simulink model "modelWithSimscapeRobotAndEnvironmentDynamics"  (R2020b)
settings: Solver=daessc  StartTime=0.0  StopTime=16  MaxStep=0.1  RelTol=1e-2  AbsTol=1e-2
values from neighbouring files (symbols this model uses):
  dq0 = zeros(size(q0))    [RobotTest.m]
  N = size(jointLim, 1)    [robotIK.m]
  q0 = homeConfiguration(lbr)    [MKC.m]    (also in RobotTest.m = configSequence(:,1))
  widgetDimensions = [0.02 0.02 0.07]    [RobotTest.m]
undefined symbols (not defined in the file or in its folder): CenterTable, configSequence, Floor, LeftShelf, X, Y, Z
libraries: sm_lib x273, nesl_utility x75, robotmaniplib x3, robotcorelib x1
(part 2 of 7)

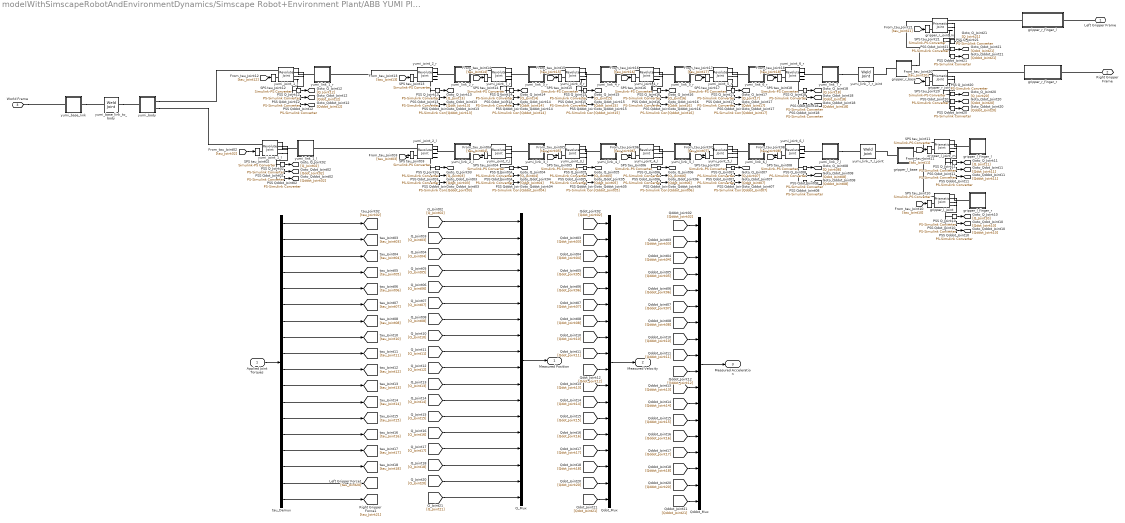
== system modelWithSimscapeRobotAndEnvironmentDynamics/Simscape Robot+Environment Plant/ABB YUMI Plant Model ==
  Applied Joint Torques : Inport
  PSS Q_Joint02 : nesl_utility/PS-Simulink Converter  PhysicalDomain=network_engine_domain  SubClassName=ps_output  LeftPortType=input  RightPortType=output  PseudoPeriodic=off  Frequencies=[]  Unit=inherit  AffineConversion=off
      settings: SourceProductName=Utilities
  PSS Q_Joint03 : nesl_utility/PS-Simulink Converter  PhysicalDomain=network_engine_domain  SubClassName=ps_output  LeftPortType=input  RightPortType=output  PseudoPeriodic=off  Frequencies=[]  Unit=inherit  AffineConversion=off
      settings: SourceProductName=Utilities
  PSS Q_Joint04 : nesl_utility/PS-Simulink Converter  PhysicalDomain=network_engine_domain  SubClassName=ps_output  LeftPortType=input  RightPortType=output  PseudoPeriodic=off  Frequencies=[]  Unit=inherit  AffineConversion=off
      settings: SourceProductName=Utilities
  PSS Q_Joint05 : nesl_utility/PS-Simulink Converter  PhysicalDomain=network_engine_domain  SubClassName=ps_output  LeftPortType=input  RightPortType=output  PseudoPeriodic=off  Frequencies=[]  Unit=inherit  AffineConversion=off
      settings: SourceProductName=Utilities
  PSS Q_Joint06 : nesl_utility/PS-Simulink Converter  PhysicalDomain=network_engine_domain  SubClassName=ps_output  LeftPortType=input  RightPortType=output  PseudoPeriodic=off  Frequencies=[]  Unit=inherit  AffineConversion=off
      settings: SourceProductName=Utilities
  PSS Q_Joint07 : nesl_utility/PS-Simulink Converter  PhysicalDomain=network_engine_domain  SubClassName=ps_output  LeftPortType=input  RightPortType=output  PseudoPeriodic=off  Frequencies=[]  Unit=inherit  AffineConversion=off
      settings: SourceProductName=Utilities
  PSS Q_Joint08 : nesl_utility/PS-Simulink Converter  PhysicalDomain=network_engine_domain  SubClassName=ps_output  LeftPortType=input  RightPortType=output  PseudoPeriodic=off  Frequencies=[]  Unit=inherit  AffineConversion=off
      settings: SourceProductName=Utilities
  PSS Q_Joint{10..18,20..21} (11 alike) : nesl_utility/PS-Simulink Converter  PhysicalDomain=network_engine_domain  SubClassName=ps_output  LeftPortType=input  RightPortType=output  PseudoPeriodic=off  Frequencies=[]  Unit=inherit  AffineConversion=off
      settings: SourceProductName=Utilities
  PSS Qddot_Joint02 : nesl_utility/PS-Simulink Converter  PhysicalDomain=network_engine_domain  SubClassName=ps_output  LeftPortType=input  RightPortType=output  PseudoPeriodic=off  Frequencies=[]  Unit=inherit  AffineConversion=off
      settings: SourceProductName=Utilities
  PSS Qddot_Joint03 : nesl_utility/PS-Simulink Converter  PhysicalDomain=network_engine_domain  SubClassName=ps_output  LeftPortType=input  RightPortType=output  PseudoPeriodic=off  Frequencies=[]  Unit=inherit  AffineConversion=off
      settings: SourceProductName=Utilities
  PSS Qddot_Joint04 : nesl_utility/PS-Simulink Converter  PhysicalDomain=network_engine_domain  SubClassName=ps_output  LeftPortType=input  RightPortType=output  PseudoPeriodic=off  Frequencies=[]  Unit=inherit  AffineConversion=off
      settings: SourceProductName=Utilities
  PSS Qddot_Joint05 : nesl_utility/PS-Simulink Converter  PhysicalDomain=network_engine_domain  SubClassName=ps_output  LeftPortType=input  RightPortType=output  PseudoPeriodic=off  Frequencies=[]  Unit=inherit  AffineConversion=off
      settings: SourceProductName=Utilities
  PSS Qddot_Joint06 : nesl_utility/PS-Simulink Converter  PhysicalDomain=network_engine_domain  SubClassName=ps_output  LeftPortType=input  RightPortType=output  PseudoPeriodic=off  Frequencies=[]  Unit=inherit  AffineConversion=off
      settings: SourceProductName=Utilities
  PSS Qddot_Joint07 : nesl_utility/PS-Simulink Converter  PhysicalDomain=network_engine_domain  SubClassName=ps_output  LeftPortType=input  RightPortType=output  PseudoPeriodic=off  Frequencies=[]  Unit=inherit  AffineConversion=off
      settings: SourceProductName=Utilities
  PSS Qddot_Joint08 : nesl_utility/PS-Simulink Converter  PhysicalDomain=network_engine_domain  SubClassName=ps_output  LeftPortType=input  RightPortType=output  PseudoPeriodic=off  Frequencies=[]  Unit=inherit  AffineConversion=off
      settings: SourceProductName=Utilities
  PSS Qddot_Joint{10..18,20..21} (11 alike) : nesl_utility/PS-Simulink Converter  PhysicalDomain=network_engine_domain  SubClassName=ps_output  LeftPortType=input  RightPortType=output  PseudoPeriodic=off  Frequencies=[]  Unit=inherit  AffineConversion=off
      settings: SourceProductName=Utilities
  PSS Qdot_Joint02 : nesl_utility/PS-Simulink Converter  PhysicalDomain=network_engine_domain  SubClassName=ps_output  LeftPortType=input  RightPortType=output  PseudoPeriodic=off  Frequencies=[]  Unit=inherit  AffineConversion=off
      settings: SourceProductName=Utilities
  PSS Qdot_Joint03 : nesl_utility/PS-Simulink Converter  PhysicalDomain=network_engine_domain  SubClassName=ps_output  LeftPortType=input  RightPortType=output  PseudoPeriodic=off  Frequencies=[]  Unit=inherit  AffineConversion=off
      settings: SourceProductName=Utilities
  PSS Qdot_Joint04 : nesl_utility/PS-Simulink Converter  PhysicalDomain=network_engine_domain  SubClassName=ps_output  LeftPortType=input  RightPortType=output  PseudoPeriodic=off  Frequencies=[]  Unit=inherit  AffineConversion=off
      settings: SourceProductName=Utilities
  PSS Qdot_Joint05 : nesl_utility/PS-Simulink Converter  PhysicalDomain=network_engine_domain  SubClassName=ps_output  LeftPortType=input  RightPortType=output  PseudoPeriodic=off  Frequencies=[]  Unit=inherit  AffineConversion=off
      settings: SourceProductName=Utilities
  PSS Qdot_Joint06 : nesl_utility/PS-Simulink Converter  PhysicalDomain=network_engine_domain  SubClassName=ps_output  LeftPortType=input  RightPortType=output  PseudoPeriodic=off  Frequencies=[]  Unit=inherit  AffineConversion=off
      settings: SourceProductName=Utilities
  PSS Qdot_Joint07 : nesl_utility/PS-Simulink Converter  PhysicalDomain=network_engine_domain  SubClassName=ps_output  LeftPortType=input  RightPortType=output  PseudoPeriodic=off  Frequencies=[]  Unit=inherit  AffineConversion=off
      settings: SourceProductName=Utilities
  PSS Qdot_Joint08 : nesl_utility/PS-Simulink Converter  PhysicalDomain=network_engine_domain  SubClassName=ps_output  LeftPortType=input  RightPortType=output  PseudoPeriodic=off  Frequencies=[]  Unit=inherit  AffineConversion=off
      settings: SourceProductName=Utilities
  PSS Qdot_Joint{10..18,20..21} (11 alike) : nesl_utility/PS-Simulink Converter  PhysicalDomain=network_engine_domain  SubClassName=ps_output  LeftPortType=input  RightPortType=output  PseudoPeriodic=off  Frequencies=[]  Unit=inherit  AffineConversion=off
      settings: SourceProductName=Utilities
  Q_Mux : Mux  Inputs=18
  Qddot_Mux : Mux  Inputs=18
  Qdot_Mux : Mux  Inputs=18
  SPS tau_Joint02 : nesl_utility/Simulink-PS Converter  PhysicalDomain=network_engine_domain  SubClassName=ps_input  LeftPortType=input  RightPortType=output  PseudoPeriodic=off  Frequencies=[]  NoiseDistribution=none  NoiseParameters=[]  Unit=1  AffineConversion=off  FilteringAndDerivatives=provide  SimscapeFilterOrder=1  InputFilterTimeConstant=0.001  UdotUserProvided=0
      settings: SourceProductName=Utilities
  SPS tau_Joint03 : nesl_utility/Simulink-PS Converter  PhysicalDomain=network_engine_domain  SubClassName=ps_input  LeftPortType=input  RightPortType=output  PseudoPeriodic=off  Frequencies=[]  NoiseDistribution=none  NoiseParameters=[]  Unit=1  AffineConversion=off  FilteringAndDerivatives=provide  SimscapeFilterOrder=1  InputFilterTimeConstant=0.001  UdotUserProvided=0
      settings: SourceProductName=Utilities
  SPS tau_Joint04 : nesl_utility/Simulink-PS Converter  PhysicalDomain=network_engine_domain  SubClassName=ps_input  LeftPortType=input  RightPortType=output  PseudoPeriodic=off  Frequencies=[]  NoiseDistribution=none  NoiseParameters=[]  Unit=1  AffineConversion=off  FilteringAndDerivatives=provide  SimscapeFilterOrder=1  InputFilterTimeConstant=0.001  UdotUserProvided=0
      settings: SourceProductName=Utilities
  SPS tau_Joint05 : nesl_utility/Simulink-PS Converter  PhysicalDomain=network_engine_domain  SubClassName=ps_input  LeftPortType=input  RightPortType=output  PseudoPeriodic=off  Frequencies=[]  NoiseDistribution=none  NoiseParameters=[]  Unit=1  AffineConversion=off  FilteringAndDerivatives=provide  SimscapeFilterOrder=1  InputFilterTimeConstant=0.001  UdotUserProvided=0
      settings: SourceProductName=Utilities
  SPS tau_Joint06 : nesl_utility/Simulink-PS Converter  PhysicalDomain=network_engine_domain  SubClassName=ps_input  LeftPortType=input  RightPortType=output  PseudoPeriodic=off  Frequencies=[]  NoiseDistribution=none  NoiseParameters=[]  Unit=1  AffineConversion=off  FilteringAndDerivatives=provide  SimscapeFilterOrder=1  InputFilterTimeConstant=0.001  UdotUserProvided=0
      settings: SourceProductName=Utilities
  SPS tau_Joint07 : nesl_utility/Simulink-PS Converter  PhysicalDomain=network_engine_domain  SubClassName=ps_input  LeftPortType=input  RightPortType=output  PseudoPeriodic=off  Frequencies=[]  NoiseDistribution=none  NoiseParameters=[]  Unit=1  AffineConversion=off  FilteringAndDerivatives=provide  SimscapeFilterOrder=1  InputFilterTimeConstant=0.001  UdotUserProvided=0
      settings: SourceProductName=Utilities
  SPS tau_Joint08 : nesl_utility/Simulink-PS Converter  PhysicalDomain=network_engine_domain  SubClassName=ps_input  LeftPortType=input  RightPortType=output  PseudoPeriodic=off  Frequencies=[]  NoiseDistribution=none  NoiseParameters=[]  Unit=1  AffineConversion=off  FilteringAndDerivatives=provide  SimscapeFilterOrder=1  InputFilterTimeConstant=0.001  UdotUserProvided=0
      settings: SourceProductName=Utilities
  SPS tau_Joint{10..18,20..21} (11 alike) : nesl_utility/Simulink-PS Converter  PhysicalDomain=network_engine_domain  SubClassName=ps_input  LeftPortType=input  RightPortType=output  PseudoPeriodic=off  Frequencies=[]  NoiseDistribution=none  NoiseParameters=[]  Unit=1  AffineConversion=off  FilteringAndDerivatives=provide  SimscapeFilterOrder=1  InputFilterTimeConstant=0.001  UdotUserProvided=0
      settings: SourceProductName=Utilities
  gripper_l_base : Subsystem
  gripper_l_finger_l : Subsystem
  gripper_l_finger_r : Subsystem
  gripper_l_joint : sm_lib/Joints/Prismatic Joint  JointMode=Normal  SenseConstraintForce=off  SenseConstraintForceX=off  SenseConstraintForceY=off  SenseConstraintForceZ=off  SenseConstraintTorque=off  SenseConstraintTorqueX=off  SenseConstraintTorqueY=off  SenseConstraintTorqueZ=off  SenseTotalForce=off  SenseTotalForceX=off  SenseTotalForceY=off  SenseTotalForceZ=off  SenseTotalTorque=off  SenseTotalTorqueX=off  SenseTotalTorqueY=off  SenseTotalTorqueZ=off  CompositeWrenchDir=FollowerOnBase  CompositeWrenchFrame=BaseFrame  EquilibriumPosition=0  EquilibriumPositionUnits=m  SpringStiffness=0  SpringStiffnessUnits=N/m  DampingCoefficient=1  DampingCoefficientUnits=kg/s  TorqueActuationMode=InputTorque  MotionActuationMode=ComputedMotion  SensePosition=on  SenseVelocity=on  SenseAcceleration=on  SenseTorqueForce=off  SenseLowerLimitTorqueForce=off  SenseUpperLimitTorqueForce=off  LowerLimitSpecify=on  LowerLimitBound=0  LowerLimitBoundUnits=m  LowerLimitStiffness=1e6  LowerLimitStiffnessUnits=N/m  LowerLimitDamping=1e3  LowerLimitDampingUnits=N/(m/s)  LowerLimitTransitionRegionWidth=1e-4  LowerLimitTransitionRegionWidthUnits=m  UpperLimitSpecify=on  UpperLimitBound=0.025  UpperLimitBoundUnits=m  UpperLimitStiffness=1e6  UpperLimitStiffnessUnits=N/m  UpperLimitDamping=1e3  UpperLimitDampingUnits=N/(m/s)  UpperLimitTransitionRegionWidth=1e-4  UpperLimitTransitionRegionWidthUnits=m  PositionTargetSpecify=on  PositionTargetPriority=High  PositionTargetValue=q0(8)  PositionTargetValueUnits=m  VelocityTargetSpecify=on  VelocityTargetPriority=High  VelocityTargetValue=dq0(8)  VelocityTargetValueUnits=m/s
      settings: SourceProductName=Multibody
  gripper_l_joint_m : sm_lib/Joints/Prismatic Joint  JointMode=Normal  SenseConstraintForce=off  SenseConstraintForceX=off  SenseConstraintForceY=off  SenseConstraintForceZ=off  SenseConstraintTorque=off  SenseConstraintTorqueX=off  SenseConstraintTorqueY=off  SenseConstraintTorqueZ=off  SenseTotalForce=off  SenseTotalForceX=off  SenseTotalForceY=off  SenseTotalForceZ=off  SenseTotalTorque=off  SenseTotalTorqueX=off  SenseTotalTorqueY=off  SenseTotalTorqueZ=off  CompositeWrenchDir=FollowerOnBase  CompositeWrenchFrame=BaseFrame  EquilibriumPosition=0  EquilibriumPositionUnits=m  SpringStiffness=0  SpringStiffnessUnits=N/m  DampingCoefficient=1  DampingCoefficientUnits=kg/s  TorqueActuationMode=InputTorque  MotionActuationMode=ComputedMotion  SensePosition=on  SenseVelocity=on  SenseAcceleration=on  SenseTorqueForce=off  SenseLowerLimitTorqueForce=off  SenseUpperLimitTorqueForce=off  LowerLimitSpecify=on  LowerLimitBound=0  LowerLimitBoundUnits=m  LowerLimitStiffness=1e6  LowerLimitStiffnessUnits=N/m  LowerLimitDamping=1e3  LowerLimitDampingUnits=N/(m/s)  LowerLimitTransitionRegionWidth=1e-4  LowerLimitTransitionRegionWidthUnits=m  UpperLimitSpecify=on  UpperLimitBound=0.025  UpperLimitBoundUnits=m  UpperLimitStiffness=1e6  UpperLimitStiffnessUnits=N/m  UpperLimitDamping=1e3  UpperLimitDampingUnits=N/(m/s)  UpperLimitTransitionRegionWidth=1e-4  UpperLimitTransitionRegionWidthUnits=m  PositionTargetSpecify=on  PositionTargetPriority=High  PositionTargetValue=q0(9)  PositionTargetValueUnits=m  VelocityTargetSpecify=on  VelocityTargetPriority=High  VelocityTargetValue=dq0(9)  VelocityTargetValueUnits=m/s
      settings: SourceProductName=Multibody
  gripper_r_base : Subsystem
  gripper_r_finger_l : Subsystem
  gripper_r_finger_r : Subsystem
  gripper_r_joint : sm_lib/Joints/Prismatic Joint  JointMode=Normal  SenseConstraintForce=off  SenseConstraintForceX=off  SenseConstraintForceY=off  SenseConstraintForceZ=off  SenseConstraintTorque=off  SenseConstraintTorqueX=off  SenseConstraintTorqueY=off  SenseConstraintTorqueZ=off  SenseTotalForce=off  SenseTotalForceX=off  SenseTotalForceY=off  SenseTotalForceZ=off  SenseTotalTorque=off  SenseTotalTorqueX=off  SenseTotalTorqueY=off  SenseTotalTorqueZ=off  CompositeWrenchDir=FollowerOnBase  CompositeWrenchFrame=BaseFrame  EquilibriumPosition=0  EquilibriumPositionUnits=m  SpringStiffness=0  SpringStiffnessUnits=N/m  DampingCoefficient=1  DampingCoefficientUnits=kg/s  TorqueActuationMode=InputTorque  MotionActuationMode=ComputedMotion  SensePosition=on  SenseVelocity=on  SenseAcceleration=on  SenseTorqueForce=off  SenseLowerLimitTorqueForce=off  SenseUpperLimitTorqueForce=off  LowerLimitSpecify=on  LowerLimitBound=0  LowerLimitBoundUnits=m  LowerLimitStiffness=1e6  LowerLimitStiffnessUnits=N/m  LowerLimitDamping=1e3  LowerLimitDampingUnits=N/(m/s)  LowerLimitTransitionRegionWidth=1e-4  LowerLimitTransitionRegionWidthUnits=m  UpperLimitSpecify=on  UpperLimitBound=0.025  UpperLimitBoundUnits=m  UpperLimitStiffness=1e6  UpperLimitStiffnessUnits=N/m  UpperLimitDamping=1e3  UpperLimitDampingUnits=N/(m/s)  UpperLimitTransitionRegionWidth=1e-4  UpperLimitTransitionRegionWidthUnits=m  PositionTargetSpecify=on  PositionTargetPriority=High  PositionTargetValue=q0(17)  PositionTargetValueUnits=m  VelocityTargetSpecify=on  VelocityTargetPriority=High  VelocityTargetValue=dq0(17)  VelocityTargetValueUnits=m/s
      settings: SourceProductName=Multibody
  gripper_r_joint_m : sm_lib/Joints/Prismatic Joint  JointMode=Normal  SenseConstraintForce=off  SenseConstraintForceX=off  SenseConstraintForceY=off  SenseConstraintForceZ=off  SenseConstraintTorque=off  SenseConstraintTorqueX=off  SenseConstraintTorqueY=off  SenseConstraintTorqueZ=off  SenseTotalForce=off  SenseTotalForceX=off  SenseTotalForceY=off  SenseTotalForceZ=off  SenseTotalTorque=off  SenseTotalTorqueX=off  SenseTotalTorqueY=off  SenseTotalTorqueZ=off  CompositeWrenchDir=FollowerOnBase  CompositeWrenchFrame=BaseFrame  EquilibriumPosition=0  EquilibriumPositionUnits=m  SpringStiffness=0  SpringStiffnessUnits=N/m  DampingCoefficient=1  DampingCoefficientUnits=kg/s  TorqueActuationMode=InputTorque  MotionActuationMode=ComputedMotion  SensePosition=on  SenseVelocity=on  SenseAcceleration=on  SenseTorqueForce=off  SenseLowerLimitTorqueForce=off  SenseUpperLimitTorqueForce=off  LowerLimitSpecify=on  LowerLimitBound=0  LowerLimitBoundUnits=m  LowerLimitStiffness=1e6  LowerLimitStiffnessUnits=N/m  LowerLimitDamping=1e3  LowerLimitDampingUnits=N/(m/s)  LowerLimitTransitionRegionWidth=1e-4  LowerLimitTransitionRegionWidthUnits=m  UpperLimitSpecify=on  UpperLimitBound=0.025  UpperLimitBoundUnits=m  UpperLimitStiffness=1e6  UpperLimitStiffnessUnits=N/m  UpperLimitDamping=1e3  UpperLimitDampingUnits=N/(m/s)  UpperLimitTransitionRegionWidth=1e-4  UpperLimitTransitionRegionWidthUnits=m  PositionTargetSpecify=on  PositionTargetPriority=High  PositionTargetValue=q0(18)  PositionTargetValueUnits=m  VelocityTargetSpecify=on  VelocityTargetPriority=High  VelocityTargetValue=dq0(18)  VelocityTargetValueUnits=m/s
      settings: SourceProductName=Multibody
  tau_Demux : Demux  Outputs=18
  yumi_base_link : Subsystem
  yumi_base_link_to_body : sm_lib/Joints/Weld Joint  JointMode=Normal  SenseConstraintForce=off  SenseConstraintForceX=off  SenseConstraintForceY=off  SenseConstraintForceZ=off  SenseConstraintTorque=off  SenseConstraintTorqueX=off  SenseConstraintTorqueY=off  SenseConstraintTorqueZ=off  SenseTotalForce=off  SenseTotalForceX=off  SenseTotalForceY=off  SenseTotalForceZ=off  SenseTotalTorque=off  SenseTotalTorqueX=off  SenseTotalTorqueY=off  SenseTotalTorqueZ=off  CompositeWrenchDir=FollowerOnBase  CompositeWrenchFrame=BaseFrame
      settings: SourceProductName=Multibody
  yumi_body : Subsystem
  yumi_joint_1_l : sm_lib/Joints/Revolute Joint  JointMode=Normal  SenseConstraintForce=off  SenseConstraintForceX=off  SenseConstraintForceY=off  SenseConstraintForceZ=off  SenseConstraintTorque=off  SenseConstraintTorqueX=off  SenseConstraintTorqueY=off  SenseConstraintTorqueZ=off  SenseTotalForce=off  SenseTotalForceX=off  SenseTotalForceY=off  SenseTotalForceZ=off  SenseTotalTorque=off  SenseTotalTorqueX=off  SenseTotalTorqueY=off  SenseTotalTorqueZ=off  CompositeWrenchDir=FollowerOnBase  CompositeWrenchFrame=BaseFrame  EquilibriumPosition=0  EquilibriumPositionUnits=deg  SpringStiffness=0  SpringStiffnessUnits=N*m/deg  DampingCoefficient=0.5  DampingCoefficientUnits=m^2*kg/s/rad  TorqueActuationMode=InputTorque  MotionActuationMode=ComputedMotion  SensePosition=on  SenseVelocity=on  SenseAcceleration=on  SenseTorqueForce=off  SenseLowerLimitTorqueForce=off  SenseUpperLimitTorqueForce=off  LowerLimitSpecify=on  LowerLimitBound=-2.94087978961  LowerLimitBoundUnits=rad  LowerLimitStiffness=1e4  LowerLimitStiffnessUnits=N*m/deg  LowerLimitDamping=10  LowerLimitDampingUnits=N*m/(deg/s)  LowerLimitTransitionRegionWidth=0.1  LowerLimitTransitionRegionWidthUnits=deg  UpperLimitSpecify=on  UpperLimitBound=2.94087978961  UpperLimitBoundUnits=rad  UpperLimitStiffness=1e4  UpperLimitStiffnessUnits=N*m/deg  UpperLimitDamping=10  UpperLimitDampingUnits=N*m/(deg/s)  UpperLimitTransitionRegionWidth=0.1  UpperLimitTransitionRegionWidthUnits=deg  PositionTargetSpecify=on  PositionTargetPriority=High  PositionTargetValue=q0(1)  PositionTargetValueUnits=rad  VelocityTargetSpecify=on  VelocityTargetPriority=High  VelocityTargetValue=dq0(1)  VelocityTargetValueUnits=rad/s
      settings: SourceProductName=Multibody
  yumi_joint_1_r : sm_lib/Joints/Revolute Joint  JointMode=Normal  SenseConstraintForce=off  SenseConstraintForceX=off  SenseConstraintForceY=off  SenseConstraintForceZ=off  SenseConstraintTorque=off  SenseConstraintTorqueX=off  SenseConstraintTorqueY=off  SenseConstraintTorqueZ=off  SenseTotalForce=off  SenseTotalForceX=off  SenseTotalForceY=off  SenseTotalForceZ=off  SenseTotalTorque=off  SenseTotalTorqueX=off  SenseTotalTorqueY=off  SenseTotalTorqueZ=off  CompositeWrenchDir=FollowerOnBase  CompositeWrenchFrame=BaseFrame  EquilibriumPosition=0  EquilibriumPositionUnits=deg  SpringStiffness=0  SpringStiffnessUnits=N*m/deg  DampingCoefficient=0.5  DampingCoefficientUnits=m^2*kg/s/rad  TorqueActuationMode=InputTorque  MotionActuationMode=ComputedMotion  SensePosition=on  SenseVelocity=on  SenseAcceleration=on  SenseTorqueForce=off  SenseLowerLimitTorqueForce=off  SenseUpperLimitTorqueForce=off  LowerLimitSpecify=on  LowerLimitBound=-2.94087978961  LowerLimitBoundUnits=rad  LowerLimitStiffness=1e4  LowerLimitStiffnessUnits=N*m/deg  LowerLimitDamping=10  LowerLimitDampingUnits=N*m/(deg/s)  LowerLimitTransitionRegionWidth=0.1  LowerLimitTransitionRegionWidthUnits=deg  UpperLimitSpecify=on  UpperLimitBound=2.94087978961  UpperLimitBoundUnits=rad  UpperLimitStiffness=1e4  UpperLimitStiffnessUnits=N*m/deg  UpperLimitDamping=10  UpperLimitDampingUnits=N*m/(deg/s)  UpperLimitTransitionRegionWidth=0.1  UpperLimitTransitionRegionWidthUnits=deg  PositionTargetSpecify=on  PositionTargetPriority=High  PositionTargetValue=q0(10)  PositionTargetValueUnits=rad  VelocityTargetSpecify=on  VelocityTargetPriority=High  VelocityTargetValue=dq0(10)  VelocityTargetValueUnits=rad/s
      settings: SourceProductName=Multibody
  yumi_joint_2_l : sm_lib/Joints/Revolute Joint  JointMode=Normal  SenseConstraintForce=off  SenseConstraintForceX=off  SenseConstraintForceY=off  SenseConstraintForceZ=off  SenseConstraintTorque=off  SenseConstraintTorqueX=off  SenseConstraintTorqueY=off  SenseConstraintTorqueZ=off  SenseTotalForce=off  SenseTotalForceX=off  SenseTotalForceY=off  SenseTotalForceZ=off  SenseTotalTorque=off  SenseTotalTorqueX=off  SenseTotalTorqueY=off  SenseTotalTorqueZ=off  CompositeWrenchDir=FollowerOnBase  CompositeWrenchFrame=BaseFrame  EquilibriumPosition=0  EquilibriumPositionUnits=deg  SpringStiffness=0  SpringStiffnessUnits=N*m/deg  DampingCoefficient=0.5  DampingCoefficientUnits=m^2*kg/s/rad  TorqueActuationMode=InputTorque  MotionActuationMode=ComputedMotion  SensePosition=on  SenseVelocity=on  SenseAcceleration=on  SenseTorqueForce=off  SenseLowerLimitTorqueForce=off  SenseUpperLimitTorqueForce=off  LowerLimitSpecify=on  LowerLimitBound=-2.50454747661  LowerLimitBoundUnits=rad  LowerLimitStiffness=1e4  LowerLimitStiffnessUnits=N*m/deg  LowerLimitDamping=10  LowerLimitDampingUnits=N*m/(deg/s)  LowerLimitTransitionRegionWidth=0.1  LowerLimitTransitionRegionWidthUnits=deg  UpperLimitSpecify=on  UpperLimitBound=0.759218224618  UpperLimitBoundUnits=rad  UpperLimitStiffness=1e4  UpperLimitStiffnessUnits=N*m/deg  UpperLimitDamping=10  UpperLimitDampingUnits=N*m/(deg/s)  UpperLimitTransitionRegionWidth=0.1  UpperLimitTransitionRegionWidthUnits=deg  PositionTargetSpecify=on  PositionTargetPriority=High  PositionTargetValue=q0(2)  PositionTargetValueUnits=rad  VelocityTargetSpecify=on  VelocityTargetPriority=High  VelocityTargetValue=dq0(2)  VelocityTargetValueUnits=rad/s
      settings: SourceProductName=Multibody
  yumi_joint_2_r : sm_lib/Joints/Revolute Joint  JointMode=Normal  SenseConstraintForce=off  SenseConstraintForceX=off  SenseConstraintForceY=off  SenseConstraintForceZ=off  SenseConstraintTorque=off  SenseConstraintTorqueX=off  SenseConstraintTorqueY=off  SenseConstraintTorqueZ=off  SenseTotalForce=off  SenseTotalForceX=off  SenseTotalForceY=off  SenseTotalForceZ=off  SenseTotalTorque=off  SenseTotalTorqueX=off  SenseTotalTorqueY=off  SenseTotalTorqueZ=off  CompositeWrenchDir=FollowerOnBase  CompositeWrenchFrame=BaseFrame  EquilibriumPosition=0  EquilibriumPositionUnits=deg  SpringStiffness=0  SpringStiffnessUnits=N*m/deg  DampingCoefficient=0.5  DampingCoefficientUnits=m^2*kg/s/rad  TorqueActuationMode=InputTorque  MotionActuationMode=ComputedMotion  SensePosition=on  SenseVelocity=on  SenseAcceleration=on  SenseTorqueForce=off  SenseLowerLimitTorqueForce=off  SenseUpperLimitTorqueForce=off  LowerLimitSpecify=on  LowerLimitBound=-2.50454747661  LowerLimitBoundUnits=rad  LowerLimitStiffness=1e4  LowerLimitStiffnessUnits=N*m/deg  LowerLimitDamping=10  LowerLimitDampingUnits=N*m/(deg/s)  LowerLimitTransitionRegionWidth=0.1  LowerLimitTransitionRegionWidthUnits=deg  UpperLimitSpecify=on  UpperLimitBound=0.759218224618  UpperLimitBoundUnits=rad  UpperLimitStiffness=1e4  UpperLimitStiffnessUnits=N*m/deg  UpperLimitDamping=10  UpperLimitDampingUnits=N*m/(deg/s)  UpperLimitTransitionRegionWidth=0.1  UpperLimitTransitionRegionWidthUnits=deg  PositionTargetSpecify=on  PositionTargetPriority=High  PositionTargetValue=q0(11)  PositionTargetValueUnits=rad  VelocityTargetSpecify=on  VelocityTargetPriority=High  VelocityTargetValue=dq0(11)  VelocityTargetValueUnits=rad/s
      settings: SourceProductName=Multibody
  yumi_joint_3_l : sm_lib/Joints/Revolute Joint  JointMode=Normal  SenseConstraintForce=off  SenseConstraintForceX=off  SenseConstraintForceY=off  SenseConstraintForceZ=off  SenseConstraintTorque=off  SenseConstraintTorqueX=off  SenseConstraintTorqueY=off  SenseConstraintTorqueZ=off  SenseTotalForce=off  SenseTotalForceX=off  SenseTotalForceY=off  SenseTotalForceZ=off  SenseTotalTorque=off  SenseTotalTorqueX=off  SenseTotalTorqueY=off  SenseTotalTorqueZ=off  CompositeWrenchDir=FollowerOnBase  CompositeWrenchFrame=BaseFrame  EquilibriumPosition=0  EquilibriumPositionUnits=deg  SpringStiffness=0  SpringStiffnessUnits=N*m/deg  DampingCoefficient=0.5  DampingCoefficientUnits=m^2*kg/s/rad  TorqueActuationMode=InputTorque  MotionActuationMode=ComputedMotion  SensePosition=on  SenseVelocity=on  SenseAcceleration=on  SenseTorqueForce=off  SenseLowerLimitTorqueForce=off  SenseUpperLimitTorqueForce=off  LowerLimitSpecify=on  LowerLimitBound=-2.15548162621  LowerLimitBoundUnits=rad  LowerLimitStiffness=1e4  LowerLimitStiffnessUnits=N*m/deg  LowerLimitDamping=10  LowerLimitDampingUnits=N*m/(deg/s)  LowerLimitTransitionRegionWidth=0.1  LowerLimitTransitionRegionWidthUnits=deg  UpperLimitSpecify=on  UpperLimitBound=1.3962634016  UpperLimitBoundUnits=rad  UpperLimitStiffness=1e4  UpperLimitStiffnessUnits=N*m/deg  UpperLimitDamping=10  UpperLimitDampingUnits=N*m/(deg/s)  UpperLimitTransitionRegionWidth=0.1  UpperLimitTransitionRegionWidthUnits=deg  PositionTargetSpecify=on  PositionTargetPriority=High  PositionTargetValue=q0(4)  PositionTargetValueUnits=rad  VelocityTargetSpecify=on  VelocityTargetPriority=High  VelocityTargetValue=dq0(4)  VelocityTargetValueUnits=rad/s
      settings: SourceProductName=Multibody
  yumi_joint_3_r : sm_lib/Joints/Revolute Joint  JointMode=Normal  SenseConstraintForce=off  SenseConstraintForceX=off  SenseConstraintForceY=off  SenseConstraintForceZ=off  SenseConstraintTorque=off  SenseConstraintTorqueX=off  SenseConstraintTorqueY=off  SenseConstraintTorqueZ=off  SenseTotalForce=off  SenseTotalForceX=off  SenseTotalForceY=off  SenseTotalForceZ=off  SenseTotalTorque=off  SenseTotalTorqueX=off  SenseTotalTorqueY=off  SenseTotalTorqueZ=off  CompositeWrenchDir=FollowerOnBase  CompositeWrenchFrame=BaseFrame  EquilibriumPosition=0  EquilibriumPositionUnits=deg  SpringStiffness=0  SpringStiffnessUnits=N*m/deg  DampingCoefficient=0.5  DampingCoefficientUnits=m^2*kg/s/rad  TorqueActuationMode=InputTorque  MotionActuationMode=ComputedMotion  SensePosition=on  SenseVelocity=on  SenseAcceleration=on  SenseTorqueForce=off  SenseLowerLimitTorqueForce=off  SenseUpperLimitTorqueForce=off  LowerLimitSpecify=on  LowerLimitBound=-2.15548162621  LowerLimitBoundUnits=rad  LowerLimitStiffness=1e4  LowerLimitStiffnessUnits=N*m/deg  LowerLimitDamping=10  LowerLimitDampingUnits=N*m/(deg/s)  LowerLimitTransitionRegionWidth=0.1  LowerLimitTransitionRegionWidthUnits=deg  UpperLimitSpecify=on  UpperLimitBound=1.3962634016  UpperLimitBoundUnits=rad  UpperLimitStiffness=1e4  UpperLimitStiffnessUnits=N*m/deg  UpperLimitDamping=10  UpperLimitDampingUnits=N*m/(deg/s)  UpperLimitTransitionRegionWidth=0.1  UpperLimitTransitionRegionWidthUnits=deg  PositionTargetSpecify=on  PositionTargetPriority=High  PositionTargetValue=q0(13)  PositionTargetValueUnits=rad  VelocityTargetSpecify=on  VelocityTargetPriority=High  VelocityTargetValue=dq0(13)  VelocityTargetValueUnits=rad/s
      settings: SourceProductName=Multibody
  yumi_joint_4_l : sm_lib/Joints/Revolute Joint  JointMode=Normal  SenseConstraintForce=off  SenseConstraintForceX=off  SenseConstraintForceY=off  SenseConstraintForceZ=off  SenseConstraintTorque=off  SenseConstraintTorqueX=off  SenseConstraintTorqueY=off  SenseConstraintTorqueZ=off  SenseTotalForce=off  SenseTotalForceX=off  SenseTotalForceY=off  SenseTotalForceZ=off  SenseTotalTorque=off  SenseTotalTorqueX=off  SenseTotalTorqueY=off  SenseTotalTorqueZ=off  CompositeWrenchDir=FollowerOnBase  CompositeWrenchFrame=BaseFrame  EquilibriumPosition=0  EquilibriumPositionUnits=deg  SpringStiffness=0  SpringStiffnessUnits=N*m/deg  DampingCoefficient=0.5  DampingCoefficientUnits=m^2*kg/s/rad  TorqueActuationMode=InputTorque  MotionActuationMode=ComputedMotion  SensePosition=on  SenseVelocity=on  SenseAcceleration=on  SenseTorqueForce=off  SenseLowerLimitTorqueForce=off  SenseUpperLimitTorqueForce=off  LowerLimitSpecify=on  LowerLimitBound=-5.06145483078  LowerLimitBoundUnits=rad  LowerLimitStiffness=1e4  LowerLimitStiffnessUnits=N*m/deg  LowerLimitDamping=10  LowerLimitDampingUnits=N*m/(deg/s)  LowerLimitTransitionRegionWidth=0.1  LowerLimitTransitionRegionWidthUnits=deg  UpperLimitSpecify=on  UpperLimitBound=5.06145483078  UpperLimitBoundUnits=rad  UpperLimitStiffness=1e4  UpperLimitStiffnessUnits=N*m/deg  UpperLimitDamping=10  UpperLimitDampingUnits=N*m/(deg/s)  UpperLimitTransitionRegionWidth=0.1  UpperLimitTransitionRegionWidthUnits=deg  PositionTargetSpecify=on  PositionTargetPriority=High  PositionTargetValue=q0(5)  PositionTargetValueUnits=rad  VelocityTargetSpecify=on  VelocityTargetPriority=High  VelocityTargetValue=dq0(5)  VelocityTargetValueUnits=rad/s
      settings: SourceProductName=Multibody
  yumi_joint_4_r : sm_lib/Joints/Revolute Joint  JointMode=Normal  SenseConstraintForce=off  SenseConstraintForceX=off  SenseConstraintForceY=off  SenseConstraintForceZ=off  SenseConstraintTorque=off  SenseConstraintTorqueX=off  SenseConstraintTorqueY=off  SenseConstraintTorqueZ=off  SenseTotalForce=off  SenseTotalForceX=off  SenseTotalForceY=off  SenseTotalForceZ=off  SenseTotalTorque=off  SenseTotalTorqueX=off  SenseTotalTorqueY=off  SenseTotalTorqueZ=off  CompositeWrenchDir=FollowerOnBase  CompositeWrenchFrame=BaseFrame  EquilibriumPosition=0  EquilibriumPositionUnits=deg  SpringStiffness=0  SpringStiffnessUnits=N*m/deg  DampingCoefficient=0.5  DampingCoefficientUnits=m^2*kg/s/rad  TorqueActuationMode=InputTorque  MotionActuationMode=ComputedMotion  SensePosition=on  SenseVelocity=on  SenseAcceleration=on  SenseTorqueForce=off  SenseLowerLimitTorqueForce=off  SenseUpperLimitTorqueForce=off  LowerLimitSpecify=on  LowerLimitBound=-5.06145483078  LowerLimitBoundUnits=rad  LowerLimitStiffness=1e4  LowerLimitStiffnessUnits=N*m/deg  LowerLimitDamping=10  LowerLimitDampingUnits=N*m/(deg/s)  LowerLimitTransitionRegionWidth=0.1  LowerLimitTransitionRegionWidthUnits=deg  UpperLimitSpecify=on  UpperLimitBound=5.06145483078  UpperLimitBoundUnits=rad  UpperLimitStiffness=1e4  UpperLimitStiffnessUnits=N*m/deg  UpperLimitDamping=10  UpperLimitDampingUnits=N*m/(deg/s)  UpperLimitTransitionRegionWidth=0.1  UpperLimitTransitionRegionWidthUnits=deg  PositionTargetSpecify=on  PositionTargetPriority=High  PositionTargetValue=q0(14)  PositionTargetValueUnits=rad  VelocityTargetSpecify=on  VelocityTargetPriority=High  VelocityTargetValue=dq0(14)  VelocityTargetValueUnits=rad/s
      settings: SourceProductName=Multibody
  yumi_joint_5_l : sm_lib/Joints/Revolute Joint  JointMode=Normal  SenseConstraintForce=off  SenseConstraintForceX=off  SenseConstraintForceY=off  SenseConstraintForceZ=off  SenseConstraintTorque=off  SenseConstraintTorqueX=off  SenseConstraintTorqueY=off  SenseConstraintTorqueZ=off  SenseTotalForce=off  SenseTotalForceX=off  SenseTotalForceY=off  SenseTotalForceZ=off  SenseTotalTorque=off  SenseTotalTorqueX=off  SenseTotalTorqueY=off  SenseTotalTorqueZ=off  CompositeWrenchDir=FollowerOnBase  CompositeWrenchFrame=BaseFrame  EquilibriumPosition=0  EquilibriumPositionUnits=deg  SpringStiffness=0  SpringStiffnessUnits=N*m/deg  DampingCoefficient=0.5  DampingCoefficientUnits=m^2*kg/s/rad  TorqueActuationMode=InputTorque  MotionActuationMode=ComputedMotion  SensePosition=on  SenseVelocity=on  SenseAcceleration=on  SenseTorqueForce=off  SenseLowerLimitTorqueForce=off  SenseUpperLimitTorqueForce=off  LowerLimitSpecify=on  LowerLimitBound=-1.53588974176  LowerLimitBoundUnits=rad  LowerLimitStiffness=1e4  LowerLimitStiffnessUnits=N*m/deg  LowerLimitDamping=10  LowerLimitDampingUnits=N*m/(deg/s)  LowerLimitTransitionRegionWidth=0.1  LowerLimitTransitionRegionWidthUnits=deg  UpperLimitSpecify=on  UpperLimitBound=2.40855436775  UpperLimitBoundUnits=rad  UpperLimitStiffness=1e4  UpperLimitStiffnessUnits=N*m/deg  UpperLimitDamping=10  UpperLimitDampingUnits=N*m/(deg/s)  UpperLimitTransitionRegionWidth=0.1  UpperLimitTransitionRegionWidthUnits=deg  PositionTargetSpecify=on  PositionTargetPriority=High  PositionTargetValue=q0(6)  PositionTargetValueUnits=rad  VelocityTargetSpecify=on  VelocityTargetPriority=High  VelocityTargetValue=dq0(6)  VelocityTargetValueUnits=rad/s
      settings: SourceProductName=Multibody
  yumi_joint_5_r : sm_lib/Joints/Revolute Joint  JointMode=Normal  SenseConstraintForce=off  SenseConstraintForceX=off  SenseConstraintForceY=off  SenseConstraintForceZ=off  SenseConstraintTorque=off  SenseConstraintTorqueX=off  SenseConstraintTorqueY=off  SenseConstraintTorqueZ=off  SenseTotalForce=off  SenseTotalForceX=off  SenseTotalForceY=off  SenseTotalForceZ=off  SenseTotalTorque=off  SenseTotalTorqueX=off  SenseTotalTorqueY=off  SenseTotalTorqueZ=off  CompositeWrenchDir=FollowerOnBase  CompositeWrenchFrame=BaseFrame  EquilibriumPosition=0  EquilibriumPositionUnits=deg  SpringStiffness=0  SpringStiffnessUnits=N*m/deg  DampingCoefficient=0.5  DampingCoefficientUnits=m^2*kg/s/rad  TorqueActuationMode=InputTorque  MotionActuationMode=ComputedMotion  SensePosition=on  SenseVelocity=on  SenseAcceleration=on  SenseTorqueForce=off  SenseLowerLimitTorqueForce=off  SenseUpperLimitTorqueForce=off  LowerLimitSpecify=on  LowerLimitBound=-1.53588974176  LowerLimitBoundUnits=rad  LowerLimitStiffness=1e4  LowerLimitStiffnessUnits=N*m/deg  LowerLimitDamping=10  LowerLimitDampingUnits=N*m/(deg/s)  LowerLimitTransitionRegionWidth=0.1  LowerLimitTransitionRegionWidthUnits=deg  UpperLimitSpecify=on  UpperLimitBound=2.40855436775  UpperLimitBoundUnits=rad  UpperLimitStiffness=1e4  UpperLimitStiffnessUnits=N*m/deg  UpperLimitDamping=10  UpperLimitDampingUnits=N*m/(deg/s)  UpperLimitTransitionRegionWidth=0.1  UpperLimitTransitionRegionWidthUnits=deg  PositionTargetSpecify=on  PositionTargetPriority=High  PositionTargetValue=q0(15)  PositionTargetValueUnits=rad  VelocityTargetSpecify=on  VelocityTargetPriority=High  VelocityTargetValue=dq0(15)  VelocityTargetValueUnits=rad/s
      settings: SourceProductName=Multibody
  yumi_joint_6_l : sm_lib/Joints/Revolute Joint  JointMode=Normal  SenseConstraintForce=off  SenseConstraintForceX=off  SenseConstraintForceY=off  SenseConstraintForceZ=off  SenseConstraintTorque=off  SenseConstraintTorqueX=off  SenseConstraintTorqueY=off  SenseConstraintTorqueZ=off  SenseTotalForce=off  SenseTotalForceX=off  SenseTotalForceY=off  SenseTotalForceZ=off  SenseTotalTorque=off  SenseTotalTorqueX=off  SenseTotalTorqueY=off  SenseTotalTorqueZ=off  CompositeWrenchDir=FollowerOnBase  CompositeWrenchFrame=BaseFrame  EquilibriumPosition=0  EquilibriumPositionUnits=deg  SpringStiffness=0  SpringStiffnessUnits=N*m/deg  DampingCoefficient=0.5  DampingCoefficientUnits=m^2*kg/s/rad  TorqueActuationMode=InputTorque  MotionActuationMode=ComputedMotion  SensePosition=on  SenseVelocity=on  SenseAcceleration=on  SenseTorqueForce=off  SenseLowerLimitTorqueForce=off  SenseUpperLimitTorqueForce=off  LowerLimitSpecify=on  LowerLimitBound=-3.99680398707  LowerLimitBoundUnits=rad  LowerLimitStiffness=1e4  LowerLimitStiffnessUnits=N*m/deg  LowerLimitDamping=10  LowerLimitDampingUnits=N*m/(deg/s)  LowerLimitTransitionRegionWidth=0.1  LowerLimitTransitionRegionWidthUnits=deg  UpperLimitSpecify=on  UpperLimitBound=3.99680398707  UpperLimitBoundUnits=rad  UpperLimitStiffness=1e4  UpperLimitStiffnessUnits=N*m/deg  UpperLimitDamping=10  UpperLimitDampingUnits=N*m/(deg/s)  UpperLimitTransitionRegionWidth=0.1  UpperLimitTransitionRegionWidthUnits=deg  PositionTargetSpecify=on  PositionTargetPriority=High  PositionTargetValue=q0(7)  PositionTargetValueUnits=rad  VelocityTargetSpecify=on  VelocityTargetPriority=High  VelocityTargetValue=dq0(7)  VelocityTargetValueUnits=rad/s
      settings: SourceProductName=Multibody
  yumi_joint_6_r : sm_lib/Joints/Revolute Joint  JointMode=Normal  SenseConstraintForce=off  SenseConstraintForceX=off  SenseConstraintForceY=off  SenseConstraintForceZ=off  SenseConstraintTorque=off  SenseConstraintTorqueX=off  SenseConstraintTorqueY=off  SenseConstraintTorqueZ=off  SenseTotalForce=off  SenseTotalForceX=off  SenseTotalForceY=off  SenseTotalForceZ=off  SenseTotalTorque=off  SenseTotalTorqueX=off  SenseTotalTorqueY=off  SenseTotalTorqueZ=off  CompositeWrenchDir=FollowerOnBase  CompositeWrenchFrame=BaseFrame  EquilibriumPosition=0  EquilibriumPositionUnits=deg  SpringStiffness=0  SpringStiffnessUnits=N*m/deg  DampingCoefficient=0.5  DampingCoefficientUnits=m^2*kg/s/rad  TorqueActuationMode=InputTorque  MotionActuationMode=ComputedMotion  SensePosition=on  SenseVelocity=on  SenseAcceleration=on  SenseTorqueForce=off  SenseLowerLimitTorqueForce=off  SenseUpperLimitTorqueForce=off  LowerLimitSpecify=on  LowerLimitBound=-3.99680398707  LowerLimitBoundUnits=rad  LowerLimitStiffness=1e4  LowerLimitStiffnessUnits=N*m/deg  LowerLimitDamping=10  LowerLimitDampingUnits=N*m/(deg/s)  LowerLimitTransitionRegionWidth=0.1  LowerLimitTransitionRegionWidthUnits=deg  UpperLimitSpecify=on  UpperLimitBound=3.99680398707  UpperLimitBoundUnits=rad  UpperLimitStiffness=1e4  UpperLimitStiffnessUnits=N*m/deg  UpperLimitDamping=10  UpperLimitDampingUnits=N*m/(deg/s)  UpperLimitTransitionRegionWidth=0.1  UpperLimitTransitionRegionWidthUnits=deg  PositionTargetSpecify=on  PositionTargetPriority=High  PositionTargetValue=q0(16)  PositionTargetValueUnits=rad  VelocityTargetSpecify=on  VelocityTargetPriority=High  VelocityTargetValue=dq0(16)  VelocityTargetValueUnits=rad/s
      settings: SourceProductName=Multibody
  yumi_joint_7_l : sm_lib/Joints/Revolute Joint  JointMode=Normal  SenseConstraintForce=off  SenseConstraintForceX=off  SenseConstraintForceY=off  SenseConstraintForceZ=off  SenseConstraintTorque=off  SenseConstraintTorqueX=off  SenseConstraintTorqueY=off  SenseConstraintTorqueZ=off  SenseTotalForce=off  SenseTotalForceX=off  SenseTotalForceY=off  SenseTotalForceZ=off  SenseTotalTorque=off  SenseTotalTorqueX=off  SenseTotalTorqueY=off  SenseTotalTorqueZ=off  CompositeWrenchDir=FollowerOnBase  CompositeWrenchFrame=BaseFrame  EquilibriumPosition=0  EquilibriumPositionUnits=deg  SpringStiffness=0  SpringStiffnessUnits=N*m/deg  DampingCoefficient=0.5  DampingCoefficientUnits=m^2*kg/s/rad  TorqueActuationMode=InputTorque  MotionActuationMode=ComputedMotion  SensePosition=on  SenseVelocity=on  SenseAcceleration=on  SenseTorqueForce=off  SenseLowerLimitTorqueForce=off  SenseUpperLimitTorqueForce=off  LowerLimitSpecify=on  LowerLimitBound=-2.94087978961  LowerLimitBoundUnits=rad  LowerLimitStiffness=1e4  LowerLimitStiffnessUnits=N*m/deg  LowerLimitDamping=10  LowerLimitDampingUnits=N*m/(deg/s)  LowerLimitTransitionRegionWidth=0.1  LowerLimitTransitionRegionWidthUnits=deg  UpperLimitSpecify=on  UpperLimitBound=2.94087978961  UpperLimitBoundUnits=rad  UpperLimitStiffness=1e4  UpperLimitStiffnessUnits=N*m/deg  UpperLimitDamping=10  UpperLimitDampingUnits=N*m/(deg/s)  UpperLimitTransitionRegionWidth=0.1  UpperLimitTransitionRegionWidthUnits=deg  PositionTargetSpecify=on  PositionTargetPriority=High  PositionTargetValue=q0(3)  PositionTargetValueUnits=rad  VelocityTargetSpecify=on  VelocityTargetPriority=High  VelocityTargetValue=dq0(3)  VelocityTargetValueUnits=rad/s
      settings: SourceProductName=Multibody
  yumi_joint_7_r : sm_lib/Joints/Revolute Joint  JointMode=Normal  SenseConstraintForce=off  SenseConstraintForceX=off  SenseConstraintForceY=off  SenseConstraintForceZ=off  SenseConstraintTorque=off  SenseConstraintTorqueX=off  SenseConstraintTorqueY=off  SenseConstraintTorqueZ=off  SenseTotalForce=off  SenseTotalForceX=off  SenseTotalForceY=off  SenseTotalForceZ=off  SenseTotalTorque=off  SenseTotalTorqueX=off  SenseTotalTorqueY=off  SenseTotalTorqueZ=off  CompositeWrenchDir=FollowerOnBase  CompositeWrenchFrame=BaseFrame  EquilibriumPosition=0  EquilibriumPositionUnits=deg  SpringStiffness=0  SpringStiffnessUnits=N*m/deg  DampingCoefficient=0.5  DampingCoefficientUnits=m^2*kg/s/rad  TorqueActuationMode=InputTorque  MotionActuationMode=ComputedMotion  SensePosition=on  SenseVelocity=on  SenseAcceleration=on  SenseTorqueForce=off  SenseLowerLimitTorqueForce=off  SenseUpperLimitTorqueForce=off  LowerLimitSpecify=on  LowerLimitBound=-2.94087978961  LowerLimitBoundUnits=rad  LowerLimitStiffness=1e4  LowerLimitStiffnessUnits=N*m/deg  LowerLimitDamping=10  LowerLimitDampingUnits=N*m/(deg/s)  LowerLimitTransitionRegionWidth=0.1  LowerLimitTransitionRegionWidthUnits=deg  UpperLimitSpecify=on  UpperLimitBound=2.94087978961  UpperLimitBoundUnits=rad  UpperLimitStiffness=1e4  UpperLimitStiffnessUnits=N*m/deg  UpperLimitDamping=10  UpperLimitDampingUnits=N*m/(deg/s)  UpperLimitTransitionRegionWidth=0.1  UpperLimitTransitionRegionWidthUnits=deg  PositionTargetSpecify=on  PositionTargetPriority=High  PositionTargetValue=q0(12)  PositionTargetValueUnits=rad  VelocityTargetSpecify=on  VelocityTargetPriority=High  VelocityTargetValue=dq0(12)  VelocityTargetValueUnits=rad/s
      settings: SourceProductName=Multibody
  yumi_link_1_l : Subsystem
  yumi_link_1_r : Subsystem
  yumi_link_2_l : Subsystem
  yumi_link_2_r : Subsystem
  yumi_link_3_l : Subsystem
  yumi_link_3_r : Subsystem
  yumi_link_4_l : Subsystem
  yumi_link_4_r : Subsystem
  yumi_link_5_l : Subsystem
  yumi_link_5_r : Subsystem
  yumi_link_6_l : Subsystem
  yumi_link_6_r : Subsystem
  yumi_link_7_l : Subsystem
  yumi_link_7_l_joint : sm_lib/Joints/Weld Joint  JointMode=Normal  SenseConstraintForce=off  SenseConstraintForceX=off  SenseConstraintForceY=off  SenseConstraintForceZ=off  SenseConstraintTorque=off  SenseConstraintTorqueX=off  SenseConstraintTorqueY=off  SenseConstraintTorqueZ=off  SenseTotalForce=off  SenseTotalForceX=off  SenseTotalForceY=off  SenseTotalForceZ=off  SenseTotalTorque=off  SenseTotalTorqueX=off  SenseTotalTorqueY=off  SenseTotalTorqueZ=off  CompositeWrenchDir=FollowerOnBase  CompositeWrenchFrame=BaseFrame
      settings: SourceProductName=Multibody
  yumi_link_7_r : Subsystem
  yumi_link_7_r_joint : sm_lib/Joints/Weld Joint  JointMode=Normal  SenseConstraintForce=off  SenseConstraintForceX=off  SenseConstraintForceY=off  SenseConstraintForceZ=off  SenseConstraintTorque=off  SenseConstraintTorqueX=off  SenseConstraintTorqueY=off  SenseConstraintTorqueZ=off  SenseTotalForce=off  SenseTotalForceX=off  SenseTotalForceY=off  SenseTotalForceZ=off  SenseTotalTorque=off  SenseTotalTorqueX=off  SenseTotalTorqueY=off  SenseTotalTorqueZ=off  CompositeWrenchDir=FollowerOnBase  CompositeWrenchFrame=BaseFrame
      settings: SourceProductName=Multibody
  Left Gripper Frame : PMIOPort  Side=Right
  Right Gripper Frame : PMIOPort  Port=2  Side=Right
  World Frame : PMIOPort  Port=3  Side=Left
  Measured Position : Outport
  Measured Velocity : Outport  Port=2
  Measured Acceleration : Outport  Port=3
  wires:
  Q_Mux/1 -> Measured Position/1
  [Qddot_Joint14] -> Qddot_Mux/12
  [Q_Joint17] -> Q_Mux/15
  tau_Demux/6 -> [tau_Joint07]
  [Qddot_Joint15] -> Qddot_Mux/13
  [Q_Joint21] -> Q_Mux/18
  PSS Q_Joint17/1 -> [Q_Joint17]
  [Qddot_Joint10] -> Qddot_Mux/8
  PSS Qddot_Joint12/1 -> [Qddot_Joint12]
  tau_Demux/13 -> [tau_Joint15]
  [Qdot_Joint18] -> Qdot_Mux/16
  PSS Qdot_Joint10/1 -> [Qdot_Joint10]
  PSS Qddot_Joint10/1 -> [Qddot_Joint10]
  [Qdot_Joint16] -> Qdot_Mux/14
  tau_Demux/3 -> [tau_Joint04]
  tau_Demux/14 -> [tau_Joint16]
  [Qddot_Joint12] -> Qddot_Mux/10
  [Qddot_Joint18] -> Qddot_Mux/16
  tau_Demux/4 -> [tau_Joint05]
  [Qddot_Joint13] -> Qddot_Mux/11
  [tau_Joint04] -> SPS tau_Joint04/1
  Applied Joint Torques/1 -> tau_Demux/1
  [tau_Joint05] -> SPS tau_Joint05/1
  [Qdot_Joint04] -> Qdot_Mux/3
  Qdot_Mux/1 -> Measured Velocity/1
  [Qdot_Joint10] -> Qdot_Mux/8
  tau_Demux/10 -> [tau_Joint12]
  PSS Q_Joint15/1 -> [Q_Joint15]
  [Qdot_Joint07] -> Qdot_Mux/6
  tau_Demux/7 -> [tau_Joint08]
  PSS Q_Joint02/1 -> [Q_Joint02]
  tau_Demux/9 -> [tau_Joint11]
  [tau_Joint21] -> SPS tau_Joint21/1
  tau_Demux/5 -> [tau_Joint06]
  [Q_Joint20] -> Q_Mux/17
  tau_Demux/1 -> [tau_Joint02]
  [Qdot_Joint17] -> Qdot_Mux/15
  [tau_Joint17] -> SPS tau_Joint17/1
  [Q_Joint05] -> Q_Mux/4
  [tau_Joint18] -> SPS tau_Joint18/1
  PSS Qddot_Joint08/1 -> [Qddot_Joint08]
  [Q_Joint02] -> Q_Mux/1
  [Qddot_Joint16] -> Qddot_Mux/14
  [Q_Joint12] -> Q_Mux/10
  PSS Qdot_Joint20/1 -> [Qdot_Joint20]
  [tau_Joint10] -> SPS tau_Joint10/1
  tau_Demux/11 -> [tau_Joint13]
  [tau_Joint07] -> SPS tau_Joint07/1
  [tau_Joint08] -> SPS tau_Joint08/1
  [tau_Joint12] -> SPS tau_Joint12/1
  PSS Qddot_Joint05/1 -> [Qddot_Joint05]
  [Qddot_Joint04] -> Qddot_Mux/3
  [Qdot_Joint15] -> Qdot_Mux/13
  [tau_Joint15] -> SPS tau_Joint15/1
  [tau_Joint03] -> SPS tau_Joint03/1
  [tau_Joint06] -> SPS tau_Joint06/1
  [Qddot_Joint20] -> Qddot_Mux/17
  [Qddot_Joint11] -> Qddot_Mux/9
  [tau_Joint02] -> SPS tau_Joint02/1
  [Qddot_Joint07] -> Qddot_Mux/6
  [tau_Joint16] -> SPS tau_Joint16/1
  tau_Demux/2 -> [tau_Joint03]
  PSS Qddot_Joint02/1 -> [Qddot_Joint02]
  [Q_Joint14] -> Q_Mux/12
  [Q_Joint15] -> Q_Mux/13
  [Q_Joint18] -> Q_Mux/16
  [Qdot_Joint11] -> Qdot_Mux/9
  [Qddot_Joint17] -> Qddot_Mux/15
  [Q_Joint16] -> Q_Mux/14
  [Q_Joint13] -> Q_Mux/11
  PSS Qddot_Joint03/1 -> [Qddot_Joint03]
  PSS Qddot_Joint15/1 -> [Qddot_Joint15]
  PSS Qddot_Joint20/1 -> [Qddot_Joint20]
  PSS Q_Joint21/1 -> [Q_Joint21]
  PSS Qddot_Joint21/1 -> [Qddot_Joint21]
  [Q_Joint10] -> Q_Mux/8
  [Q_Joint06] -> Q_Mux/5
  PSS Qddot_Joint18/1 -> [Qddot_Joint18]
  tau_Demux/12 -> [tau_Joint14]
  PSS Q_Joint20/1 -> [Q_Joint20]
  PSS Qdot_Joint18/1 -> [Qdot_Joint18]
  [Qdot_Joint05] -> Qdot_Mux/4
  [Q_Joint08] -> Q_Mux/7
  PSS Q_Joint11/1 -> [Q_Joint11]
  PSS Qdot_Joint15/1 -> [Qdot_Joint15]
  PSS Qdot_Joint12/1 -> [Qdot_Joint12]
  PSS Q_Joint14/1 -> [Q_Joint14]
  tau_Demux/16 -> [tau_Joint18]
  [Q_Joint11] -> Q_Mux/9
  PSS Q_Joint08/1 -> [Q_Joint08]
  tau_Demux/18 -> [tau_Joint21]
  PSS Qddot_Joint13/1 -> [Qddot_Joint13]
  [Qddot_Joint05] -> Qddot_Mux/4
  PSS Qddot_Joint17/1 -> [Qddot_Joint17]
  PSS Q_Joint05/1 -> [Q_Joint05]
  Qddot_Mux/1 -> Measured Acceleration/1
  [tau_Joint20] -> SPS tau_Joint20/1
  PSS Qdot_Joint06/1 -> [Qdot_Joint06]
  PSS Qdot_Joint17/1 -> [Qdot_Joint17]
  PSS Q_Joint13/1 -> [Q_Joint13]
  [Qdot_Joint06] -> Qdot_Mux/5
  [Qddot_Joint02] -> Qddot_Mux/1
  tau_Demux/8 -> [tau_Joint10]
  [Q_Joint03] -> Q_Mux/2
  PSS Qdot_Joint14/1 -> [Qdot_Joint14]
  PSS Qdot_Joint21/1 -> [Qdot_Joint21]
  PSS Q_Joint03/1 -> [Q_Joint03]
  PSS Qddot_Joint07/1 -> [Qddot_Joint07]
  [Qdot_Joint14] -> Qdot_Mux/12
  [Qddot_Joint03] -> Qddot_Mux/2
  PSS Q_Joint06/1 -> [Q_Joint06]
  tau_Demux/17 -> [tau_Joint20]
  PSS Q_Joint18/1 -> [Q_Joint18]
  [tau_Joint11] -> SPS tau_Joint11/1
  [Qdot_Joint02] -> Qdot_Mux/1
  tau_Demux/15 -> [tau_Joint17]
  [tau_Joint14] -> SPS tau_Joint14/1
  [Qddot_Joint21] -> Qddot_Mux/18
  PSS Qdot_Joint03/1 -> [Qdot_Joint03]
  [Q_Joint04] -> Q_Mux/3
  PSS Qdot_Joint08/1 -> [Qdot_Joint08]
  PSS Qdot_Joint13/1 -> [Qdot_Joint13]
  [Qdot_Joint20] -> Qdot_Mux/17
  [Qdot_Joint12] -> Qdot_Mux/10
  PSS Qddot_Joint14/1 -> [Qddot_Joint14]
  PSS Qdot_Joint16/1 -> [Qdot_Joint16]
  [Qdot_Joint21] -> Qdot_Mux/18
  [Qdot_Joint03] -> Qdot_Mux/2
  [Qddot_Joint06] -> Qddot_Mux/5
  PSS Qdot_Joint02/1 -> [Qdot_Joint02]
  PSS Q_Joint16/1 -> [Q_Joint16]
  PSS Qdot_Joint11/1 -> [Qdot_Joint11]
  PSS Q_Joint10/1 -> [Q_Joint10]
  PSS Q_Joint04/1 -> [Q_Joint04]
  PSS Qdot_Joint07/1 -> [Qdot_Joint07]
  PSS Q_Joint07/1 -> [Q_Joint07]
  [Qdot_Joint08] -> Qdot_Mux/7
  PSS Qddot_Joint06/1 -> [Qddot_Joint06]
  PSS Qddot_Joint04/1 -> [Qddot_Joint04]
  PSS Qdot_Joint05/1 -> [Qdot_Joint05]
  [Q_Joint07] -> Q_Mux/6
  [tau_Joint13] -> SPS tau_Joint13/1
  PSS Qddot_Joint11/1 -> [Qddot_Joint11]
  PSS Q_Joint12/1 -> [Q_Joint12]
  PSS Qdot_Joint04/1 -> [Qdot_Joint04]
  [Qddot_Joint08] -> Qddot_Mux/7
  PSS Qddot_Joint16/1 -> [Qddot_Joint16]
  [Qdot_Joint13] -> Qdot_Mux/11
  connections:
  yumi_joint_6_r/RConn2 -- PSS Q_Joint18/LConn1
  SPS tau_Joint17/RConn1 -- yumi_joint_5_r/LConn2
  yumi_link_7_l/RConn1 -- yumi_link_7_l_joint/LConn1
  yumi_joint_3_l/RConn1 -- yumi_link_4_l/LConn1
  yumi_joint_7_l/RConn1 -- yumi_link_3_l/LConn1
  SPS tau_Joint04/RConn1 -- yumi_joint_7_l/LConn2
  yumi_joint_4_l/RConn2 -- PSS Q_Joint06/LConn1
  yumi_joint_6_r/LConn1 -- yumi_link_6_r/RConn1
  yumi_joint_5_r/RConn1 -- yumi_link_6_r/LConn1
  yumi_joint_5_l/RConn4 -- PSS Qddot_Joint07/LConn1
  yumi_joint_2_l/RConn3 -- PSS Qdot_Joint03/LConn1
  yumi_joint_3_l/LConn1 -- yumi_link_3_l/RConn1
  SPS tau_Joint18/RConn1 -- yumi_joint_6_r/LConn2
  yumi_joint_1_r/RConn4 -- PSS Qddot_Joint12/LConn1
  gripper_l_base/LConn1 -- yumi_link_7_l_joint/RConn1
  SPS tau_Joint10/RConn1 -- gripper_l_joint/LConn2
  SPS tau_Joint20/RConn1 -- gripper_r_joint/LConn2
  SPS tau_Joint14/RConn1 -- yumi_joint_7_r/LConn2
  yumi_joint_6_l/RConn1 -- yumi_link_7_l/LConn1
  gripper_l_base/RConn2 -- gripper_l_joint/LConn1
  SPS tau_Joint16/RConn1 -- yumi_joint_4_r/LConn2
  SPS tau_Joint11/RConn1 -- gripper_l_joint_m/LConn2
  SPS tau_Joint03/RConn1 -- yumi_joint_2_l/LConn2
  SPS tau_Joint07/RConn1 -- yumi_joint_5_l/LConn2
  gripper_l_joint_m/RConn2 -- PSS Q_Joint11/LConn1
  SPS tau_Joint13/RConn1 -- yumi_joint_2_r/LConn2
  yumi_joint_5_r/RConn3 -- PSS Qdot_Joint17/LConn1
  yumi_joint_1_l/RConn1 -- yumi_link_1_l/LConn1
  yumi_joint_7_r/RConn4 -- PSS Qddot_Joint14/LConn1
  SPS tau_Joint21/RConn1 -- gripper_r_joint_m/LConn2
  SPS tau_Joint12/RConn1 -- yumi_joint_1_r/LConn2
  yumi_joint_3_r/RConn1 -- yumi_link_4_r/LConn1
  yumi_joint_5_r/LConn1 -- yumi_link_5_r/RConn1
  gripper_r_joint_m/RConn4 -- PSS Qddot_Joint21/LConn1
  gripper_r_joint_m/RConn2 -- PSS Q_Joint21/LConn1
  gripper_l_finger_r/LConn1 -- gripper_l_joint/RConn1
  yumi_joint_4_r/RConn4 -- PSS Qddot_Joint16/LConn1
  yumi_joint_4_r/RConn3 -- PSS Qdot_Joint16/LConn1
  SPS tau_Joint06/RConn1 -- yumi_joint_4_l/LConn2
  yumi_joint_4_l/RConn1 -- yumi_link_5_l/LConn1
  yumi_joint_7_r/RConn3 -- PSS Qdot_Joint14/LConn1
  yumi_joint_4_r/RConn2 -- PSS Q_Joint16/LConn1
  yumi_joint_2_l/LConn1 -- yumi_link_1_l/RConn1
  yumi_joint_1_l/RConn2 -- PSS Q_Joint02/LConn1
  SPS tau_Joint15/RConn1 -- yumi_joint_3_r/LConn2
  yumi_joint_7_l/RConn2 -- PSS Q_Joint04/LConn1
  yumi_joint_3_r/RConn2 -- PSS Q_Joint15/LConn1
  yumi_body/RConn2 -- yumi_joint_1_l/LConn1
  gripper_r_joint/RConn2 -- PSS Q_Joint20/LConn1
  yumi_joint_3_r/RConn3 -- PSS Qdot_Joint15/LConn1
  yumi_joint_2_l/RConn2 -- PSS Q_Joint03/LConn1
  yumi_joint_2_l/RConn1 -- yumi_link_2_l/LConn1
  yumi_joint_1_l/RConn4 -- PSS Qddot_Joint02/LConn1
  yumi_joint_2_r/RConn1 -- yumi_link_2_r/LConn1
  yumi_joint_3_l/RConn2 -- PSS Q_Joint05/LConn1
  yumi_joint_4_r/LConn1 -- yumi_link_4_r/RConn1
  yumi_joint_6_l/LConn1 -- yumi_link_6_l/RConn1
  yumi_joint_3_r/RConn4 -- PSS Qddot_Joint15/LConn1
  yumi_joint_5_l/LConn1 -- yumi_link_5_l/RConn1
  yumi_joint_6_r/RConn1 -- yumi_link_7_r/LConn1
  SPS tau_Joint05/RConn1 -- yumi_joint_3_l/LConn2
  yumi_joint_7_r/RConn1 -- yumi_link_3_r/LConn1
  gripper_r_joint/RConn3 -- PSS Qdot_Joint20/LConn1
  yumi_joint_6_r/RConn3 -- PSS Qdot_Joint18/LConn1
  yumi_joint_1_r/RConn1 -- yumi_link_1_r/LConn1
  SPS tau_Joint08/RConn1 -- yumi_joint_6_l/LConn2
  gripper_r_joint/RConn4 -- PSS Qddot_Joint20/LConn1
  yumi_joint_6_l/RConn2 -- PSS Q_Joint08/LConn1
  yumi_joint_2_r/LConn1 -- yumi_link_1_r/RConn1
  gripper_l_joint/RConn3 -- PSS Qdot_Joint10/LConn1
  yumi_joint_4_l/RConn4 -- PSS Qddot_Joint06/LConn1
  gripper_r_base/LConn1 -- yumi_link_7_r_joint/RConn1
  Left Gripper Frame/RConn1 -- gripper_r_finger_l/RConn1
  yumi_body/RConn1 -- yumi_joint_1_r/LConn1
  gripper_l_joint/RConn2 -- PSS Q_Joint10/LConn1
  yumi_joint_7_r/RConn2 -- PSS Q_Joint14/LConn1
  yumi_joint_1_r/RConn3 -- PSS Qdot_Joint12/LConn1
  yumi_joint_2_r/RConn4 -- PSS Qddot_Joint13/LConn1
  gripper_l_joint_m/RConn3 -- PSS Qdot_Joint11/LConn1
  yumi_joint_2_r/RConn3 -- PSS Qdot_Joint13/LConn1
  yumi_joint_1_r/RConn2 -- PSS Q_Joint12/LConn1
  gripper_l_joint_m/RConn4 -- PSS Qddot_Joint11/LConn1
  gripper_r_base/RConn2 -- gripper_r_joint/LConn1
  yumi_joint_7_l/LConn1 -- yumi_link_2_l/RConn1
  yumi_joint_2_r/RConn2 -- PSS Q_Joint13/LConn1
  yumi_joint_4_r/RConn1 -- yumi_link_5_r/LConn1
  yumi_joint_3_l/RConn4 -- PSS Qddot_Joint05/LConn1
  yumi_joint_5_r/RConn2 -- PSS Q_Joint17/LConn1
  yumi_joint_6_l/RConn3 -- PSS Qdot_Joint08/LConn1
  yumi_joint_5_l/RConn2 -- PSS Q_Joint07/LConn1
  yumi_joint_5_l/RConn3 -- PSS Qdot_Joint07/LConn1
  yumi_joint_3_l/RConn3 -- PSS Qdot_Joint05/LConn1
  yumi_joint_7_l/RConn3 -- PSS Qdot_Joint04/LConn1
  yumi_joint_4_l/RConn3 -- PSS Qdot_Joint06/LConn1
  yumi_joint_6_l/RConn4 -- PSS Qddot_Joint08/LConn1
  yumi_joint_2_l/RConn4 -- PSS Qddot_Joint03/LConn1
  yumi_joint_5_r/RConn4 -- PSS Qddot_Joint17/LConn1
  yumi_joint_7_l/RConn4 -- PSS Qddot_Joint04/LConn1
  gripper_r_base/RConn1 -- gripper_r_joint_m/LConn1
  yumi_joint_6_r/RConn4 -- PSS Qddot_Joint18/LConn1
  yumi_joint_1_l/RConn3 -- PSS Qdot_Joint02/LConn1
  yumi_base_link_to_body/RConn1 -- yumi_body/LConn1
  yumi_joint_7_r/LConn1 -- yumi_link_2_r/RConn1
  Right Gripper Frame/RConn1 -- gripper_r_finger_r/RConn1
  yumi_joint_5_l/RConn1 -- yumi_link_6_l/LConn1
  gripper_l_finger_l/LConn1 -- gripper_l_joint_m/RConn1
  yumi_link_7_r/RConn1 -- yumi_link_7_r_joint/LConn1
  gripper_l_joint/RConn4 -- PSS Qddot_Joint10/LConn1
  yumi_joint_4_l/LConn1 -- yumi_link_4_l/RConn1
  gripper_r_joint_m/RConn3 -- PSS Qdot_Joint21/LConn1
  yumi_joint_3_r/LConn1 -- yumi_link_3_r/RConn1
  SPS tau_Joint02/RConn1 -- yumi_joint_1_l/LConn2
  yumi_base_link/RConn1 -- yumi_base_link_to_body/LConn1
  gripper_l_base/RConn1 -- gripper_l_joint_m/LConn1
  gripper_r_finger_l/LConn1 -- gripper_r_joint_m/RConn1
  gripper_r_finger_r/LConn1 -- gripper_r_joint/RConn1
  World Frame/RConn1 -- yumi_base_link/LConn1
